simulink model "untitled1"  (R2024b)
settings: Solver=VariableStepAuto  StartTime=0.0  StopTime=10.0  RelTol=1e-3
undefined symbols (not defined in the file or in its folder): b, J, K, L, R, Vin
settings Model: Creator=aminh  LastModifiedBy=aminh

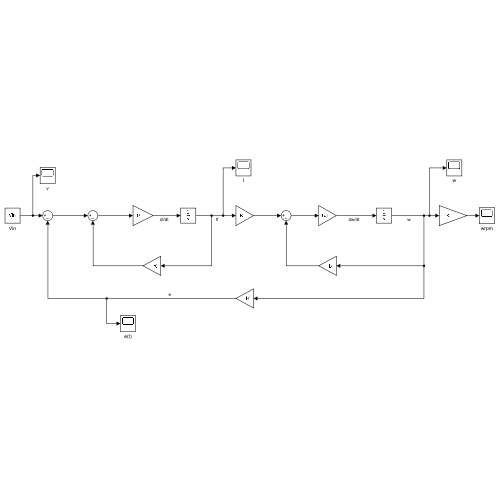
[thumbnail: Simulink's stored preview of the top-level diagram]
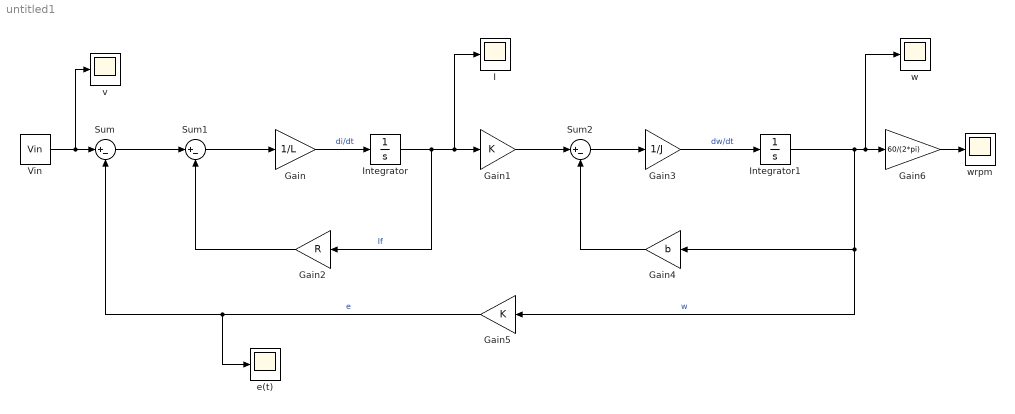
== system untitled1 ==
  Gain : Gain  Gain=1/L
  Gain1 : Gain  Gain=K
  Gain2 : Gain  Gain=R
  Gain3 : Gain  Gain=1/J
  Gain4 : Gain  Gain=b
  Gain5 : Gain  Gain=K
  Gain6 : Gain  Gain=60/(2*pi)
  I : Scope
  Integrator : Integrator
  Integrator1 : Integrator
  Sum : Sum  Inputs=|+-
  Sum1 : Sum  Inputs=|+-
  Sum2 : Sum  Inputs=|+-
  Vin : Constant  Value=Vin
  e(t) : Scope
  v : Scope
  w : Scope
  wrpm : Scope
  wires:
  Vin/1 -> v/1, Sum/1
  Integrator/1 -> Gain2/1, I/1, Gain1/1  "If"
  Gain3/1 -> Integrator1/1  "dw/dt"
  Sum1/1 -> Gain/1
  Sum2/1 -> Gain3/1
  Gain4/1 -> Sum2/2
  Gain/1 -> Integrator/1  "di/dt"
  Gain5/1 -> e(t)/1, Sum/2  "e"
  Gain2/1 -> Sum1/2
  Gain1/1 -> Sum2/1
  Sum/1 -> Sum1/1
  Gain6/1 -> wrpm/1
  Integrator1/1 -> w/1, Gain6/1, Gain5/1, Gain4/1  "w"
